simulink model "traj_test_sa_1"  (R2013b)
settings: Solver=ode4  StartTime=0.0  StopTime=4  FixedStep=0.001  RelTol=1e-3
(part 1 of 3)
settings Model: Creator=lucius  LastModifiedBy=lucius
settings DataIOCC: LimitDataPoints=off

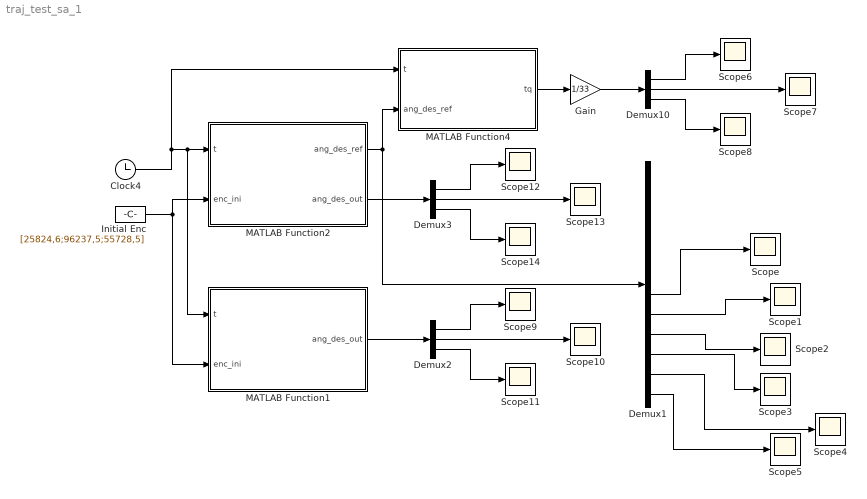
== system traj_test_sa_1 ==
  Clock4 : Clock
  Demux1 : Demux  Outputs=12
  Demux10 : Demux  Outputs=3
  Demux2 : Demux  Outputs=3
  Demux3 : Demux  Outputs=3
  Gain : Gain  Gain=1/33
  Initial Enc : Constant  Value=[25824,6;96237,5;55728,5]
  MATLAB Function1 : MATLAB Function  TreatAsAtomicUnit=on
  MATLAB Function2 : MATLAB Function  TreatAsAtomicUnit=on
  MATLAB Function4 : MATLAB Function  TreatAsAtomicUnit=on
  Scope{,1..14} (15 alike) : Scope
      Scope10 settings: SaveName=ScopeData9
      Scope11 settings: SaveName=ScopeData10
      Scope12 settings: SaveName=ScopeData12
      Scope13 settings: SaveName=ScopeData13
      Scope14 settings: SaveName=ScopeData14
      Scope2 settings: SaveName=ScopeData2
      Scope3 settings: SaveName=ScopeData3
      Scope4 settings: SaveName=ScopeData4
      Scope5 settings: SaveName=ScopeData5
      Scope6 settings: SaveName=ScopeData6
      Scope7 settings: SaveName=ScopeData7
      Scope8 settings: SaveName=ScopeData8
      Scope9 settings: SaveName=ScopeData11
  wires:
  Initial Enc/1 -> MATLAB Function2/2(enc_ini), MATLAB Function1/2(enc_ini)
  MATLAB Function2/1(ang_des_ref) -> Demux1/1, MATLAB Function4/2(ang_des_ref)
  Demux10/1 -> Scope6/1
  Demux10/2 -> Scope7/1
  Demux10/3 -> Scope8/1
  Gain/1 -> Demux10/1
  MATLAB Function4/1(tq) -> Gain/1
  Demux1/12 -> Scope5/1
  Demux1/11 -> Scope4/1
  Demux1/10 -> Scope3/1
  Demux1/7 -> Scope/1
  Demux1/8 -> Scope1/1
  Demux1/9 -> Scope2/1
  Clock4/1 -> MATLAB Function4/1(t), MATLAB Function1/1(t), MATLAB Function2/1(t)
  Demux2/1 -> Scope9/1
  Demux2/2 -> Scope10/1
  Demux2/3 -> Scope11/1
  MATLAB Function1/1(ang_des_out) -> Demux2/1
  Demux3/1 -> Scope12/1
  Demux3/2 -> Scope13/1
  Demux3/3 -> Scope14/1
  MATLAB Function2/2(ang_des_out) -> Demux3/1
